simulink model "MIT_normalized"  (R2021a)
settings: Solver=VariableStepAuto  StartTime=0.0  StopTime=400  RelTol=1e-3
values from neighbouring files (symbols this model uses):
  a0 = 1/(tau1*tau2)    (= 1.4940706006e-05)    [TA1.m]
  a0m = 10    [TA1.m]
  a1 = (tau1+tau2+A*R2)/(tau1*tau2)    (= 0.0166321059812)    [TA1.m]
  a1m = 14    [TA1.m]
  alpha = 0.001    [TA1.m]
  b = R2/(tau1*tau2)    (= 1.64347766066e-05)    [TA1.m]
  gamma = 3000    [TA1.m]
settings Model: Creator=ASUS  LastModifiedBy=ASUS

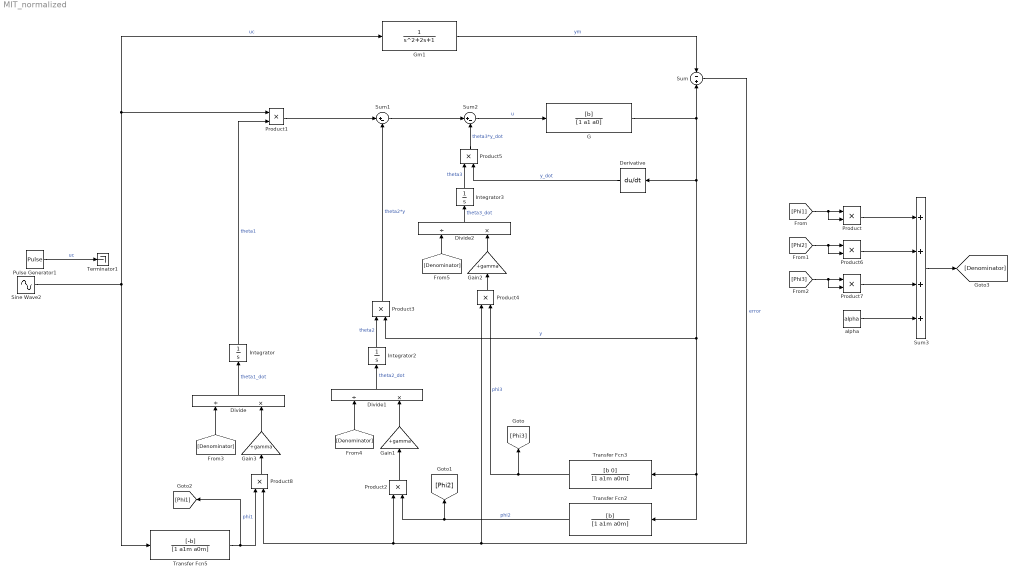
== system MIT_normalized ==
  Derivative : Derivative
  Divide : Product  Inputs=/*
  Divide1 : Product  Inputs=/*
  Divide2 : Product  Inputs=/*
  G : TransferFcn  Numerator=[b]  Denominator=[1 a1 a0]
  Gain1 : Gain  Gain=+gamma
  Gain2 : Gain  Gain=+gamma
  Gain3 : Gain  Gain=+gamma
  Gm1 : TransferFcn
  Integrator : Integrator
  Integrator2 : Integrator
  Integrator3 : Integrator
  Product{,1..8} (9 alike) : Product
  Pulse Generator1 : DiscretePulseGenerator  PulseType=Time based  Period=100  PulseWidth=50
  Sine Wave2 : Sin  Amplitude=10  Frequency=0.1  SampleTime=0
  Sum : Sum  Inputs=-+
  Sum1 : Sum  Inputs=|+-
  Sum2 : Sum  Inputs=|+-
  Sum3 : Sum  Inputs=++++
  Terminator1 : Terminator
  Transfer Fcn2 : TransferFcn  Numerator=[b]  Denominator=[1 a1m a0m]
  Transfer Fcn3 : TransferFcn  Numerator=[b 0]  Denominator=[1 a1m a0m]
  Transfer Fcn5 : TransferFcn  Numerator=[-b]  Denominator=[1 a1m a0m]
  alpha : Constant  Value=alpha
  wires:
  Sum1/1 -> Sum2/1
  Integrator2/1 -> Product3/1  "theta2"
  Gm1/1 -> Sum/1  "ym"
  Derivative/1 -> Product5/2  "y_dot"
  Product2/1 -> Gain1/1
  Sum2/1 -> G/1  "u"
  Sum/1 -> Product4/1, Product2/1, Product8/2  "error"
  Product5/1 -> Sum2/2  "theta3*y_dot"
  Product3/1 -> Sum1/2  "theta2*y"
  G/1 -> Sum/2, Transfer Fcn2/1, Transfer Fcn3/1, Product3/2, Derivative/1  "y"
  Product1/1 -> Sum1/1
  Integrator3/1 -> Product5/1  "theta3"
  Sine Wave2/1 -> Transfer Fcn5/1, Gm1/1, Product1/1  "uc"
  Product4/1 -> Gain2/1
  Transfer Fcn3/1 -> Product4/2, [Phi3]  "phi3"
  Transfer Fcn2/1 -> Product2/2, [Phi2]  "phi2"
  Transfer Fcn5/1 -> Product8/1, [Phi1]  "phi1"
  [Phi1] -> Product/2, Product/1
  [Phi2] -> Product6/2, Product6/1
  [Phi3] -> Product7/2, Product7/1
  Product/1 -> Sum3/1
  Product6/1 -> Sum3/2
  Product7/1 -> Sum3/3
  alpha/1 -> Sum3/4
  Sum3/1 -> [Denominator]
  Product8/1 -> Gain3/1
  Gain3/1 -> Divide/2
  [Denominator] -> Divide/1
  Divide/1 -> Integrator/1  "theta1_dot"
  Integrator/1 -> Product1/2  "theta1"
  [Denominator] -> Divide1/1
  Gain1/1 -> Divide1/2
  Divide1/1 -> Integrator2/1  "theta2_dot"
  [Denominator] -> Divide2/1
  Gain2/1 -> Divide2/2
  Divide2/1 -> Integrator3/1  "theta3_dot"
  Pulse Generator1/1 -> Terminator1/1  "uc"
